simulink model "simulink_shoulder"  (R2024b)
settings: Solver=VariableStepAuto  StartTime=0.0  StopTime=3  FixedStep=0.02  RelTol=1e-3  AbsTol=1e-3  EnableMultiTasking=on
InitFcn:
  | main;
values from neighbouring files (symbols this model uses):
  initEul = params.InitPosOptEul.initCondEul    [simulink_main.m]
  initQuat = params.InitPosOptEul.initCondQuat    [simulink_main.m]
  model = das3_readosim(osim_file,['Motions\',motion_name,'\',polyfiles_dir,'\',musclepoly_file])    [create_files.m]    (also in das3_polynomials.m = das3_readosim(osimfile); matlab.mat = ; plot_results.m = load(OS_model); simulink_main.m = params.model)
  N = 10000    [trials.m]
  s = fx.getSize()    [das3_readosim.m]
undefined symbols (not defined in the file or in its folder): initSimScape, X, Y, Z
libraries: sm_lib x47, nesl_utility x22
(part 2 of 2)

== system simulink_shoulder/Simscape model/Scapula ==
  body : sm_lib/Body Elements/File Solid  ExtGeomFileName=Geometry/rscapula_mod.obj  UnitType=Custom  ExtGeomFileUnits=m  StepReaderType=HEX  ExportConvexHullGeometry=off  InertiaType=Custom  BasedOnType=Density  Density=1850  DensityUnits=kg/m^3  Mass=model.mass_scapula  MassUnits=kg  CenterOfMass=model.com_scapula  CenterOfMassUnits=m  MomentsOfInertia=model.I_scapula(1:3)  MomentsOfInertiaUnits=kg*m^2  ProductsOfInertia=model.I_scapula(4:6)  ProductsOfInertiaUnits=kg*m^2  GraphicType=FromGeometry  MarkerShape=Sphere  MarkerSize=10  GraphicVisPropType=SimpleVisualProperties  GraphicDiffuseColor=[0.5 0.5 0.5]  GraphicOpacity=1.0  GraphicSpecularColor=[0.5 0.5 0.5 1.0]  GraphicAmbientColor=[0.15 0.15 0.15 1.0]  GraphicEmissiveColor=[0.0 0.0 0.0 1.0]  GraphicShininess=75  DoExposeReferenceFrame=on  SerializedFrames=<Frames><Frame><Id>Frame1</Id><Value><Name>COM</Name><Origin><Source>CenterOfMassFrame</Source><FeatureName></FeatureName></Origin><PrimaryAxis><DefinedDirection>+Z</DefinedDirection><Source>ReferenceFrame</Source><SourceDirection>+Z</SourceDirection><FeatureName></FeatureName></PrimaryAxis><SecondaryAxis><DefinedDirection>+X</DefinedDirection><Source>ReferenceFrame</Source><SourceDirection>+X</SourceDirection><FeatureName></FeatureName></SecondaryAxis></Value></Frame></Frames>
  CoM : PMIOPort  Side=Right
  connections:
  CoM/RConn1 -- body/LConn1

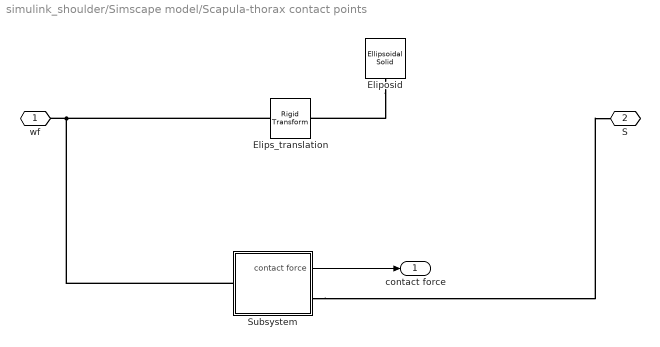
== system simulink_shoulder/Simscape model/Scapula-thorax contact points ==
  Eliposid : sm_lib/Body Elements/Ellipsoidal Solid  EllipsoidRadii=model.elips_dim*model.first_elips_scale  EllipsoidRadiiUnits=m  ExportEntireGeometry=off  InertiaType=PointMass  BasedOnType=Density  Density=1000  DensityUnits=kg/m^3  Mass=0.001  MassUnits=kg  CenterOfMass=[0 0 0]  CenterOfMassUnits=m  MomentsOfInertia=[1 1 1]  MomentsOfInertiaUnits=kg*m^2  ProductsOfInertia=[0 0 0]  ProductsOfInertiaUnits=kg*m^2  GraphicType=FromGeometry  MarkerShape=Sphere  MarkerSize=10  GraphicVisPropType=SimpleVisualProperties  GraphicDiffuseColor=[1 0 0]  GraphicOpacity=0.2  GraphicSpecularColor=[0.5 0.5 0.5 1.0]  GraphicAmbientColor=[0.15 0.15 0.15 1.0]  GraphicEmissiveColor=[0.0 0.0 0.0 1.0]  GraphicShininess=75  DoExposeReferenceFrame=on  SerializedFrames=<Frames/>
  Elips_translation : sm_lib/Frames and Transforms/Rigid Transform  RotationMethod=None  FollAlignAxisA=+X  BaseAlignAxisA=+Y  FollAlignAxisB=+Y  BaseAlignAxisB=+Z  RotationStandardAxis=+Z  RotationAngle=0.0  RotationAngleUnits=deg  RotationArbitraryAxis=[0 0 1]  RotationSequenceAxes=FollowerAxes  RotationSequence=XYX  RotationSequenceAngles=[0 0 0]  RotationSequenceAnglesUnits=deg  RotationMatrix=[1 0 0; 0 1 0; 0 0 1]  Quaternion=[1 0 0 0]  TranslationMethod=Cartesian  TranslationCartesianOffset=model.elips_trans  TranslationCartesianOffsetUnits=m  TranslationStandardAxis=+Z  TranslationStandardOffset=0  TranslationStandardOffsetUnits=m  TranslationROffset=0  TranslationROffsetUnits=m  TranslationThetaOffset=0  TranslationThetaOffsetUnits=deg  TranslationZOffset=0  TranslationZOffsetUnits=m
  Subsystem : Subsystem
  wf : PMIOPort  Side=Left
  S : PMIOPort  Port=2  Side=Right
  contact force : Outport
  wires:
  Subsystem/1(contact force) -> contact force/1
  connections:
  Elips_translation/LConn1 -- Subsystem/LConn1 -- wf/RConn1
  Subsystem/RConn1 -- S/RConn1
  Eliposid/RConn1 -- Elips_translation/RConn1

== system simulink_shoulder/Simscape model/Ulna ==
  body : sm_lib/Body Elements/File Solid  ExtGeomFileName=Geometry/rulna_transformed.obj  UnitType=Custom  ExtGeomFileUnits=m  StepReaderType=HEX  ExportConvexHullGeometry=off  InertiaType=Custom  BasedOnType=Density  Density=1850  DensityUnits=kg/m^3  Mass=model.mass_ulna  MassUnits=kg  CenterOfMass=model.com_ulna  CenterOfMassUnits=m  MomentsOfInertia=model.I_ulna(1:3)  MomentsOfInertiaUnits=kg*m^2  ProductsOfInertia=model.I_ulna(4:6)  ProductsOfInertiaUnits=kg*m^2  GraphicType=FromGeometry  MarkerShape=Sphere  MarkerSize=10  GraphicVisPropType=SimpleVisualProperties  GraphicDiffuseColor=[0.5 0.5 0.5]  GraphicOpacity=1.0  GraphicSpecularColor=[0.5 0.5 0.5 1.0]  GraphicAmbientColor=[0.15 0.15 0.15 1.0]  GraphicEmissiveColor=[0.0 0.0 0.0 1.0]  GraphicShininess=75  DoExposeReferenceFrame=on  SerializedFrames=<Frames><Frame><Id>Frame1</Id><Value><Name>F1</Name><Origin><Source>CenterOfMassFrame</Source><FeatureName></FeatureName></Origin><PrimaryAxis><DefinedDirection>+Z</DefinedDirection><Source>ReferenceFrame</Source><SourceDirection>+Z</SourceDirection><FeatureName></FeatureName></PrimaryAxis><SecondaryAxis><DefinedDirection>+X</DefinedDirection><Source>ReferenceFrame</Source><SourceDirection>+X</SourceDirection><FeatureName></FeatureName></SecondaryAxis></Value></Frame></Frames>
  CoM : PMIOPort  Side=Left
  connections:
  body/LConn1 -- CoM/RConn1

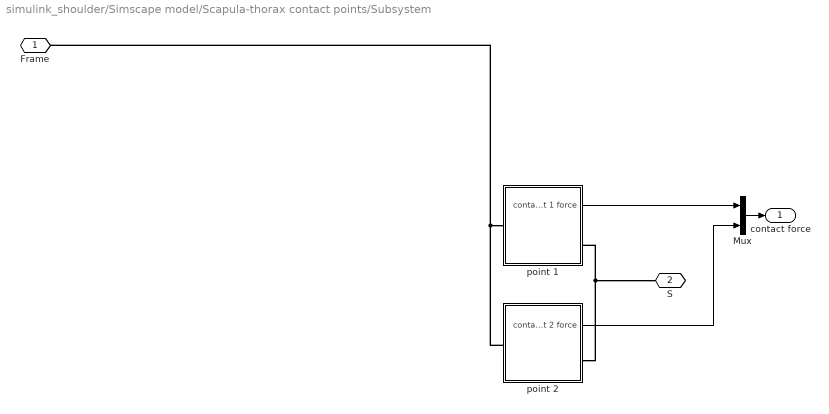
== system simulink_shoulder/Simscape model/Scapula-thorax contact points/Subsystem ==
  Mux : Mux  Inputs=2
  point 1 : Subsystem
  point 2 : Subsystem
  Frame : PMIOPort  Side=Left
  S : PMIOPort  Port=2  Side=Right
  contact force : Outport
  wires:
  point 2/1(contact point 2 force) -> Mux/2
  point 1/1(contact point 1 force) -> Mux/1
  Mux/1 -> contact force/1
  connections:
  point 2/LConn1 -- Frame/RConn1 -- point 1/LConn1
  point 2/RConn1 -- point 1/RConn1 -- S/RConn1

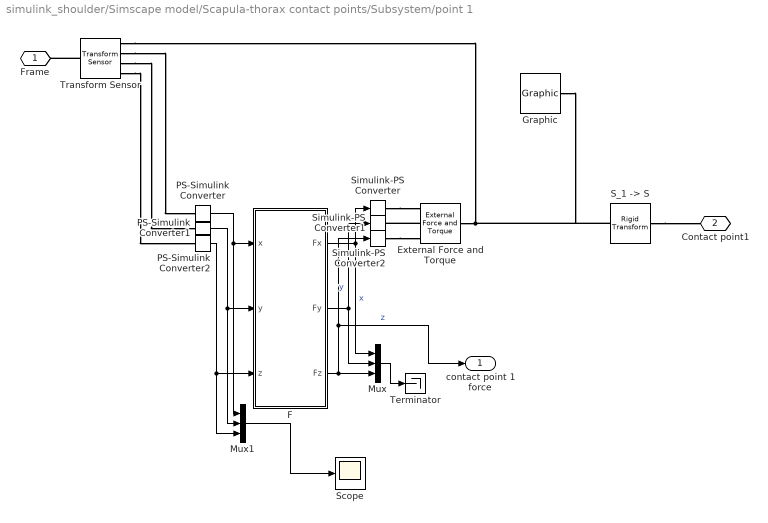
== system simulink_shoulder/Simscape model/Scapula-thorax contact points/Subsystem/point 1 ==
  External Force and Torque : sm_lib/Forces and Torques/External Force and Torque  EnableForceX=on  EnableForceY=on  EnableForceZ=on  EnableForce=off  ForceResolutionFrame=World  EnableTorqueX=off  EnableTorqueY=off  EnableTorqueZ=off  EnableTorque=off  TorqueResolutionFrame=AttachedFrame
  F : MATLAB Function  TreatAsAtomicUnit=on
  Graphic : sm_lib/Body Elements/Graphic  GraphicType=Marker  MarkerShape=Sphere  MarkerSize=10  GraphicVisPropType=SimpleVisualProperties  GraphicDiffuseColor=[0 1 0]  GraphicOpacity=1.0  GraphicSpecularColor=[0.5 0.5 0.5 1.0]  GraphicAmbientColor=[0.15 0.15 0.15 1.0]  GraphicEmissiveColor=[0.0 0.0 0.0 1.0]  GraphicShininess=75
  Mux : Mux  Inputs=3
  Mux1 : Mux  Inputs=3
  PS-Simulink Converter : nesl_utility/PS-Simulink Converter  PhysicalDomain=network_engine_domain  SubClassName=ps_output  LeftPortType=input  RightPortType=output  PseudoPeriodic=off  Frequencies=[]  VectorFormat=inherit  Unit=inherit  AffineConversion=off
  PS-Simulink Converter1 : nesl_utility/PS-Simulink Converter  PhysicalDomain=network_engine_domain  SubClassName=ps_output  LeftPortType=input  RightPortType=output  PseudoPeriodic=off  Frequencies=[]  VectorFormat=inherit  Unit=inherit  AffineConversion=off
  PS-Simulink Converter2 : nesl_utility/PS-Simulink Converter  PhysicalDomain=network_engine_domain  SubClassName=ps_output  LeftPortType=input  RightPortType=output  PseudoPeriodic=off  Frequencies=[]  VectorFormat=inherit  Unit=inherit  AffineConversion=off
  "S_1 -> S" : sm_lib/Frames and Transforms/Rigid Transform  RotationMethod=None  FollAlignAxisA=+X  BaseAlignAxisA=+Y  FollAlignAxisB=+Y  BaseAlignAxisB=+Z  RotationStandardAxis=+Z  RotationAngle=0.0  RotationAngleUnits=deg  RotationArbitraryAxis=[0 0 1]  RotationSequenceAxes=FollowerAxes  RotationSequence=XYX  RotationSequenceAngles=[0 0 0]  RotationSequenceAnglesUnits=deg  RotationMatrix=[1 0 0; 0 1 0; 0 0 1]  Quaternion=[1 0 0 0]  TranslationMethod=Cartesian  TranslationCartesianOffset=model.contTS  TranslationCartesianOffsetUnits=m  TranslationStandardAxis=+Z  TranslationStandardOffset=0  TranslationStandardOffsetUnits=m  TranslationROffset=0  TranslationROffsetUnits=m  TranslationThetaOffset=0  TranslationThetaOffsetUnits=deg  TranslationZOffset=0  TranslationZOffsetUnits=m
  Scope : Scope
  Simulink-PS Converter : nesl_utility/Simulink-PS Converter  PhysicalDomain=network_engine_domain  SubClassName=ps_input  LeftPortType=input  RightPortType=output  PseudoPeriodic=off  Frequencies=[]  NoiseDistribution=none  NoiseParameters=[]  Unit=1  AffineConversion=off  FilteringAndDerivatives=provide  SimscapeFilterOrder=1  InputFilterTimeConstant=0.001  UdotUserProvided=0
  Simulink-PS Converter1 : nesl_utility/Simulink-PS Converter  PhysicalDomain=network_engine_domain  SubClassName=ps_input  LeftPortType=input  RightPortType=output  PseudoPeriodic=off  Frequencies=[]  NoiseDistribution=none  NoiseParameters=[]  Unit=1  AffineConversion=off  FilteringAndDerivatives=provide  SimscapeFilterOrder=1  InputFilterTimeConstant=0.001  UdotUserProvided=0
  Simulink-PS Converter2 : nesl_utility/Simulink-PS Converter  PhysicalDomain=network_engine_domain  SubClassName=ps_input  LeftPortType=input  RightPortType=output  PseudoPeriodic=off  Frequencies=[]  NoiseDistribution=none  NoiseParameters=[]  Unit=1  AffineConversion=off  FilteringAndDerivatives=provide  SimscapeFilterOrder=1  InputFilterTimeConstant=0.001  UdotUserProvided=0
  Terminator : Terminator
  Transform Sensor : sm_lib/Frames and Transforms/Transform Sensor  MeasurementFrame=World  RotationSequence=XYX  SenseAngle=off  SenseAxis=off  SenseQ=off  SenseR=off  SenseRotationSequence=off  SenseOmegaX=off  SenseOmegaY=off  SenseOmegaZ=off  SenseOmega=off  SenseQDot=off  SenseRDot=off  SenseRotationSequenceDot=off  SenseAlphaX=off  SenseAlphaY=off  SenseAlphaZ=off  SenseAlpha=off  SenseQDDot=off  SenseRDDot=off  SenseX=on  SenseY=on  SenseZ=on  SenseXYZ=off  SenseRad=off  SenseAzim=off  SenseDist=off  SenseInc=off  SenseXDot=off  SenseYDot=off  SenseZDot=off  SenseXYZDot=off  SenseRadDot=off  SenseAzimDot=off  SenseDistDot=off  SenseIncDot=off  SenseXDDot=off  SenseYDDot=off  SenseZDDot=off  SenseXYZDDot=off  SenseRadDDot=off  SenseAzimDDot=off  SenseDistDDot=off  SenseIncDDot=off
  Frame : PMIOPort  Side=Left
  Contact point1 : PMIOPort  Port=2  Side=Right
  contact point 1 force : Outport
  wires:
  PS-Simulink Converter2/1 -> Mux1/3, F/3(z)
  F/3(Fz) -> contact point 1 force/1, Simulink-PS Converter2/1, Mux/3  "z"
  PS-Simulink Converter1/1 -> Mux1/2, F/2(y)
  F/1(Fx) -> Simulink-PS Converter/1, Mux/1  "x"
  F/2(Fy) -> Simulink-PS Converter1/1, Mux/2  "y"
  PS-Simulink Converter/1 -> Mux1/1, F/1(x)
  Mux1/1 -> Scope/1
  Mux/1 -> Terminator/1
  connections:
  External Force and Torque/LConn2 -- Simulink-PS Converter1/RConn1
  Transform Sensor/RConn4 -- PS-Simulink Converter2/LConn1
  Transform Sensor/RConn2 -- PS-Simulink Converter/LConn1
  Transform Sensor/LConn1 -- Frame/RConn1
  Simulink-PS Converter/RConn1 -- External Force and Torque/LConn1
  Transform Sensor/RConn3 -- PS-Simulink Converter1/LConn1
  Simulink-PS Converter2/RConn1 -- External Force and Torque/LConn3
  External Force and Torque/RConn1 -- Graphic/RConn1 -- "S_1 -> S"/RConn1 -- Transform Sensor/RConn1
  "S_1 -> S"/LConn1 -- Contact point1/RConn1

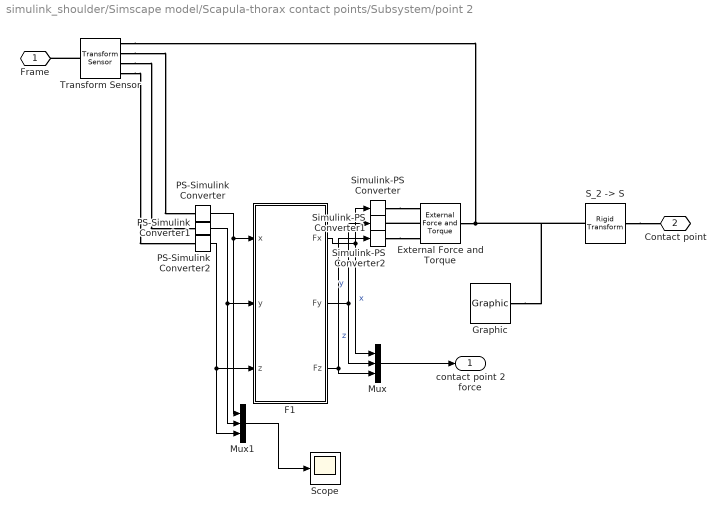
== system simulink_shoulder/Simscape model/Scapula-thorax contact points/Subsystem/point 2 ==
  External Force and Torque : sm_lib/Forces and Torques/External Force and Torque  EnableForceX=on  EnableForceY=on  EnableForceZ=on  EnableForce=off  ForceResolutionFrame=World  EnableTorqueX=off  EnableTorqueY=off  EnableTorqueZ=off  EnableTorque=off  TorqueResolutionFrame=AttachedFrame
  F1 : MATLAB Function  TreatAsAtomicUnit=on
  Graphic : sm_lib/Body Elements/Graphic  GraphicType=Marker  MarkerShape=Sphere  MarkerSize=10  GraphicVisPropType=SimpleVisualProperties  GraphicDiffuseColor=[0 1 0]  GraphicOpacity=1.0  GraphicSpecularColor=[0.5 0.5 0.5 1.0]  GraphicAmbientColor=[0.15 0.15 0.15 1.0]  GraphicEmissiveColor=[0.0 0.0 0.0 1.0]  GraphicShininess=75
  Mux : Mux  Inputs=3
  Mux1 : Mux  Inputs=3
  PS-Simulink Converter : nesl_utility/PS-Simulink Converter  PhysicalDomain=network_engine_domain  SubClassName=ps_output  LeftPortType=input  RightPortType=output  PseudoPeriodic=off  Frequencies=[]  VectorFormat=inherit  Unit=inherit  AffineConversion=off
  PS-Simulink Converter1 : nesl_utility/PS-Simulink Converter  PhysicalDomain=network_engine_domain  SubClassName=ps_output  LeftPortType=input  RightPortType=output  PseudoPeriodic=off  Frequencies=[]  VectorFormat=inherit  Unit=inherit  AffineConversion=off
  PS-Simulink Converter2 : nesl_utility/PS-Simulink Converter  PhysicalDomain=network_engine_domain  SubClassName=ps_output  LeftPortType=input  RightPortType=output  PseudoPeriodic=off  Frequencies=[]  VectorFormat=inherit  Unit=inherit  AffineConversion=off
  "S_2 -> S" : sm_lib/Frames and Transforms/Rigid Transform  RotationMethod=None  FollAlignAxisA=+X  BaseAlignAxisA=+Y  FollAlignAxisB=+Y  BaseAlignAxisB=+Z  RotationStandardAxis=+Z  RotationAngle=0.0  RotationAngleUnits=deg  RotationArbitraryAxis=[0 0 1]  RotationSequenceAxes=FollowerAxes  RotationSequence=XYX  RotationSequenceAngles=[0 0 0]  RotationSequenceAnglesUnits=deg  RotationMatrix=[1 0 0; 0 1 0; 0 0 1]  Quaternion=[1 0 0 0]  TranslationMethod=Cartesian  TranslationCartesianOffset=model.contAI  TranslationCartesianOffsetUnits=m  TranslationStandardAxis=+Z  TranslationStandardOffset=0  TranslationStandardOffsetUnits=m  TranslationROffset=0  TranslationROffsetUnits=m  TranslationThetaOffset=0  TranslationThetaOffsetUnits=deg  TranslationZOffset=0  TranslationZOffsetUnits=m
  Scope : Scope
  Simulink-PS Converter : nesl_utility/Simulink-PS Converter  PhysicalDomain=network_engine_domain  SubClassName=ps_input  LeftPortType=input  RightPortType=output  PseudoPeriodic=off  Frequencies=[]  NoiseDistribution=none  NoiseParameters=[]  Unit=1  AffineConversion=off  FilteringAndDerivatives=provide  SimscapeFilterOrder=1  InputFilterTimeConstant=0.001  UdotUserProvided=0
  Simulink-PS Converter1 : nesl_utility/Simulink-PS Converter  PhysicalDomain=network_engine_domain  SubClassName=ps_input  LeftPortType=input  RightPortType=output  PseudoPeriodic=off  Frequencies=[]  NoiseDistribution=none  NoiseParameters=[]  Unit=1  AffineConversion=off  FilteringAndDerivatives=provide  SimscapeFilterOrder=1  InputFilterTimeConstant=0.001  UdotUserProvided=0
  Simulink-PS Converter2 : nesl_utility/Simulink-PS Converter  PhysicalDomain=network_engine_domain  SubClassName=ps_input  LeftPortType=input  RightPortType=output  PseudoPeriodic=off  Frequencies=[]  NoiseDistribution=none  NoiseParameters=[]  Unit=1  AffineConversion=off  FilteringAndDerivatives=provide  SimscapeFilterOrder=1  InputFilterTimeConstant=0.001  UdotUserProvided=0
  Transform Sensor : sm_lib/Frames and Transforms/Transform Sensor  MeasurementFrame=World  RotationSequence=XYX  SenseAngle=off  SenseAxis=off  SenseQ=off  SenseR=off  SenseRotationSequence=off  SenseOmegaX=off  SenseOmegaY=off  SenseOmegaZ=off  SenseOmega=off  SenseQDot=off  SenseRDot=off  SenseRotationSequenceDot=off  SenseAlphaX=off  SenseAlphaY=off  SenseAlphaZ=off  SenseAlpha=off  SenseQDDot=off  SenseRDDot=off  SenseX=on  SenseY=on  SenseZ=on  SenseXYZ=off  SenseRad=off  SenseAzim=off  SenseDist=off  SenseInc=off  SenseXDot=off  SenseYDot=off  SenseZDot=off  SenseXYZDot=off  SenseRadDot=off  SenseAzimDot=off  SenseDistDot=off  SenseIncDot=off  SenseXDDot=off  SenseYDDot=off  SenseZDDot=off  SenseXYZDDot=off  SenseRadDDot=off  SenseAzimDDot=off  SenseDistDDot=off  SenseIncDDot=off
  Frame : PMIOPort  Side=Left
  Contact point : PMIOPort  Port=2  Side=Right
  contact point 2 force : Outport
  wires:
  PS-Simulink Converter/1 -> F1/1(x), Mux1/1
  F1/2(Fy) -> Simulink-PS Converter1/1, Mux/2  "y"
  F1/1(Fx) -> Mux/1, Simulink-PS Converter/1  "x"
  PS-Simulink Converter1/1 -> F1/2(y), Mux1/2
  Mux/1 -> contact point 2 force/1
  F1/3(Fz) -> Simulink-PS Converter2/1, Mux/3  "z"
  PS-Simulink Converter2/1 -> F1/3(z), Mux1/3
  Mux1/1 -> Scope/1
  connections:
  Transform Sensor/RConn1 -- Graphic/RConn1 -- "S_2 -> S"/RConn1 -- External Force and Torque/RConn1
  Simulink-PS Converter2/RConn1 -- External Force and Torque/LConn3
  Transform Sensor/RConn3 -- PS-Simulink Converter1/LConn1
  Simulink-PS Converter/RConn1 -- External Force and Torque/LConn1
  Transform Sensor/LConn1 -- Frame/RConn1
  Transform Sensor/RConn2 -- PS-Simulink Converter/LConn1
  Transform Sensor/RConn4 -- PS-Simulink Converter2/LConn1
  External Force and Torque/LConn2 -- Simulink-PS Converter1/RConn1
  "S_2 -> S"/LConn1 -- Contact point/RConn1

== matlab function simulink_shoulder/Simscape model/Conoid ligmanet/MATLAB Function ==
  data: l input; F output; d output; model parameter
function [F,d] = fcn(l,model)
lopt = model.conoid_length;
k = model.conoid_stiffness;
eps = model.conoid_eps;
d = l-lopt;
F = -k/2*(d+sqrt(d^2+eps));

== matlab function simulink_shoulder/Simscape model/Scapula-thorax contact points/Subsystem/point 1/F ==
  data: x input; Fx output; y input; z input; Fy output; Fz output; model parameter
function [Fx,Fy,Fz]= fcn(x,y,z,model)

f_in = ((x-model.elips_trans(1))/(model.first_elips_scale*model.elips_dim(1)))^2+((y-model.elips_trans(2))/(model.first_elips_scale*model.elips_dim(2)))^2+((z-model.elips_trans(3))/(model.first_elips_scale*model.elips_dim(3)))^2-1;
f_out = ((x-model.elips_trans(1))/(model.second_elips_scale*model.elips_dim(1)))^2+((y-model.elips_trans(2))/(model.second_elips_scale*model.elips_dim(2)))^2+((z-model.elips_trans(3))/(model.second_elips_scale*model.elips_dim(3)))^2-1;
F_in = 1/2*(f_in-sqrt(f_in^2+model.eps_in^2));
F_out = 1/2*(f_out+sqrt(f_out^2+model.eps_out^2));

Fx = -(model.k_contact_in*F_in+model.k_contact_out*F_out)*(x-model.elips_trans(1))*(model.elips_dim(1)^2+model.elips_dim(2)^2+model.elips_dim(3)^2)/(model.elips_dim(1)^2);
Fy = -(model.k_contact_in*F_in+model.k_contact_out*F_out)*(y-model.elips_trans(2))*(model.elips_dim(1)^2+model.elips_dim(2)^2+model.elips_dim(3)^2)/(model.elips_dim(2)^2);
Fz = -(model.k_contact_in*F_in+model.k_contact_out*F_out)*(z-model.elips_trans(3))*(model.elips_dim(1)^2+model.elips_dim(2)^2+model.elips_dim(3)^2)/(model.elips_dim(3)^2);

%% 2D
% 
% f = ((x-mx)/model.elips_dim(1))^2+((z-mz)/model.elips_dim(3))^2-1;
% F = 1/2*(f-sqrt(f^2+eps^2));
% 
% Fx = -k*(x-mx)*(model.elips_dim(1)^2+model.elips_dim(2)^2)/(model.elips_dim(1)^2)*F;
% Fy = -k*(y-my)*(model.elips_dim(1)^2+model.elips_dim(2)^2)/(model.elips_dim(2)^2)*F;
% Fz = -k*(z-mz)*(model.elips_dim(1)^2+model.elips_dim(2)^2)/(model.elips_dim(3)^2)*F;

== matlab function simulink_shoulder/Simscape model/Scapula-thorax contact points/Subsystem/point 2/F1 ==
  data: x input; Fx output; y input; z input; Fy output; Fz output; model parameter
function [Fx,Fy,Fz]= fcn(x,y,z,model)

f_in = ((x-model.elips_trans(1))/(model.first_elips_scale*model.elips_dim(1)))^2+((y-model.elips_trans(2))/(model.first_elips_scale*model.elips_dim(2)))^2+((z-model.elips_trans(3))/(model.first_elips_scale*model.elips_dim(3)))^2-1;
f_out = ((x-model.elips_trans(1))/(model.second_elips_scale*model.elips_dim(1)))^2+((y-model.elips_trans(2))/(model.second_elips_scale*model.elips_dim(2)))^2+((z-model.elips_trans(3))/(model.second_elips_scale*model.elips_dim(3)))^2-1;
F_in = 1/2*(f_in-sqrt(f_in^2+model.eps_in^2));
F_out = 1/2*(f_out+sqrt(f_out^2+model.eps_out^2));

Fx = -(model.k_contact_in*F_in+model.k_contact_out*F_out)*(x-model.elips_trans(1))*(model.elips_dim(1)^2+model.elips_dim(2)^2+model.elips_dim(3)^2)/(model.elips_dim(1)^2);
Fy = -(model.k_contact_in*F_in+model.k_contact_out*F_out)*(y-model.elips_trans(2))*(model.elips_dim(1)^2+model.elips_dim(2)^2+model.elips_dim(3)^2)/(model.elips_dim(2)^2);
Fz = -(model.k_contact_in*F_in+model.k_contact_out*F_out)*(z-model.elips_trans(3))*(model.elips_dim(1)^2+model.elips_dim(2)^2+model.elips_dim(3)^2)/(model.elips_dim(3)^2);

%% 2D
% 
% f = ((x-mx)/model.elips_dim(1))^2+((z-mz)/model.elips_dim(3))^2-1;
% F = 1/2*(f-sqrt(f^2+eps^2));
% 
% Fx = -k*(x-mx)*(model.elips_dim(1)^2+model.elips_dim(2)^2)/(model.elips_dim(1)^2)*F;
% Fy = -k*(y-my)*(model.elips_dim(1)^2+model.elips_dim(2)^2)/(model.elips_dim(2)^2)*F;
% Fz = -k*(z-mz)*(model.elips_dim(1)^2+model.elips_dim(2)^2)/(model.elips_dim(3)^2)*F;

== matlab function simulink_shoulder/Euler angles-based model ==
  data: x input; model parameter; y output; qSC output; qAC output; qGH output; qulna output
function [y,qSC,qAC,qGH,qulna] = fcn(x,model)
qSC = x(1:3);
qAC = x(4:6);
qGH = x(7:9);
qulna = x(10);
t = 0;
y = zeros(20,1);
mm = mm_eul(t,x(1:10),x(11:20),model); % space-joint mass matrix
fo = fo_eul(t,x(1:10),x(11:20),model); % external forces
TE_conoid = TE_conoid_eul(0,x(1:10),model); % conoid ligamentum
y = mm\(fo+[zeros(10,1);TE_conoid']);

== matlab function simulink_shoulder/Quaternion-based model ==
  data: x input; y output; qSC output; qAC output; qGH output; qulna output; model parameter
function [y,qSC,qAC,qGH,qulna] = fcn(x,model)
y = zeros(23,1);
q1 = x(1:4);
q2 = x(5:8);
q3 = x(9:12);
q4 = x(13);

% renormalize quaternions
q1new = q1/norm(q1);
q2new = q2/norm(q2);
q3new = q3/norm(q2);
u = x(14:end);
t = 0;
qSC = q1new;
qAC = q2new;
qGH = q3new;
qulna = q4;

mm = mm_quat(t,[q1new;q2new;q3new;x(13)],u,model); % space-joint mass matrix
fo = fo_quat(t,[q1new;q2new;q3new;x(13)],u,model); % external forces
TE_conoid = [zeros(13,1);TE_conoid_quat(t,[q1new;q2new;q3new;x(13)],model)']; %conoid ligamentum
y = mm\(fo+TE_conoid);

end
